simulink model "qn"  (R2025b)
settings: Solver=ode4  StartTime=0.0  StopTime=85  FixedStep=0.001  RelTol=1e-3
InitFcn:
  | % Codex-added defaults for qn controller parameters.
(part 2 of 2)

== system qn/11/control/eh uav pd10/Subsystem9 ==
  u : Inport
  MATLAB Function17 : MATLAB Function  TreatAsAtomicUnit=on
  y : Outport
  wires:
  u/1 -> MATLAB Function17/2(u)
  MATLAB Function17/1(y) -> y/1
  [falg] -> MATLAB Function17/1(flag)

== system qn/11/control/eh uav pd2/Subsystem1 ==
  u : Inport
  MATLAB Function15 : MATLAB Function  TreatAsAtomicUnit=on
  y : Outport
  wires:
  MATLAB Function15/1(y) -> y/1
  u/1 -> MATLAB Function15/2(u)
  [falg] -> MATLAB Function15/1(flag)

== system qn/11/control/eh uav pd2/Subsystem12 ==
  u : Inport
  MATLAB Function15 : MATLAB Function  TreatAsAtomicUnit=on
  y : Outport
  wires:
  MATLAB Function15/1(y) -> y/1
  u/1 -> MATLAB Function15/2(u)
  [falg] -> MATLAB Function15/1(flag)

== system qn/11/control/eh uav pd2/Subsystem2 ==
  u : Inport
  MATLAB Function15 : MATLAB Function  TreatAsAtomicUnit=on
  y : Outport
  wires:
  MATLAB Function15/1(y) -> y/1
  u/1 -> MATLAB Function15/2(u)
  [falg] -> MATLAB Function15/1(flag)

== system qn/11/control/eh uav pd3/Subsystem1 ==
  u : Inport
  MATLAB Function15 : MATLAB Function  TreatAsAtomicUnit=on
  y : Outport
  wires:
  MATLAB Function15/1(y) -> y/1
  u/1 -> MATLAB Function15/2(u)
  [falg] -> MATLAB Function15/1(flag)

== system qn/11/control/eh uav pd3/Subsystem12 ==
  u : Inport
  MATLAB Function15 : MATLAB Function  TreatAsAtomicUnit=on
  y : Outport
  wires:
  MATLAB Function15/1(y) -> y/1
  u/1 -> MATLAB Function15/2(u)
  [falg] -> MATLAB Function15/1(flag)

== system qn/11/control/eh uav pd3/Subsystem2 ==
  u : Inport
  MATLAB Function15 : MATLAB Function  TreatAsAtomicUnit=on
  y : Outport
  wires:
  MATLAB Function15/1(y) -> y/1
  u/1 -> MATLAB Function15/2(u)
  [falg] -> MATLAB Function15/1(flag)

== system qn/11/control/eh uav pd4/Subsystem1 ==
  u : Inport
  MATLAB Function15 : MATLAB Function  TreatAsAtomicUnit=on
  y : Outport
  wires:
  MATLAB Function15/1(y) -> y/1
  u/1 -> MATLAB Function15/2(u)
  [falg] -> MATLAB Function15/1(flag)

== system qn/11/control/eh uav pd4/Subsystem12 ==
  u : Inport
  MATLAB Function15 : MATLAB Function  TreatAsAtomicUnit=on
  y : Outport
  wires:
  MATLAB Function15/1(y) -> y/1
  u/1 -> MATLAB Function15/2(u)
  [falg] -> MATLAB Function15/1(flag)

== system qn/11/control/eh uav pd4/Subsystem2 ==
  u : Inport
  MATLAB Function15 : MATLAB Function  TreatAsAtomicUnit=on
  y : Outport
  wires:
  MATLAB Function15/1(y) -> y/1
  u/1 -> MATLAB Function15/2(u)
  [falg] -> MATLAB Function15/1(flag)

== system qn/11/control/eh uav pd5/Subsystem1 ==
  u : Inport
  MATLAB Function15 : MATLAB Function  TreatAsAtomicUnit=on
  y : Outport
  wires:
  MATLAB Function15/1(y) -> y/1
  u/1 -> MATLAB Function15/2(u)
  [falg] -> MATLAB Function15/1(flag)

== system qn/11/control/eh uav pd5/Subsystem12 ==
  u : Inport
  MATLAB Function15 : MATLAB Function  TreatAsAtomicUnit=on
  y : Outport
  wires:
  MATLAB Function15/1(y) -> y/1
  u/1 -> MATLAB Function15/2(u)
  [falg] -> MATLAB Function15/1(flag)

== system qn/11/control/eh uav pd5/Subsystem2 ==
  u : Inport
  MATLAB Function15 : MATLAB Function  TreatAsAtomicUnit=on
  y : Outport
  wires:
  MATLAB Function15/1(y) -> y/1
  u/1 -> MATLAB Function15/2(u)
  [falg] -> MATLAB Function15/1(flag)

== system qn/11/control/eh uav pd6/Subsystem1 ==
  u : Inport
  MATLAB Function17 : MATLAB Function  TreatAsAtomicUnit=on
  y : Outport
  wires:
  u/1 -> MATLAB Function17/2(u)
  MATLAB Function17/1(y) -> y/1
  [falg] -> MATLAB Function17/1(flag)

== system qn/11/control/eh uav pd6/Subsystem2 ==
  u : Inport
  MATLAB Function17 : MATLAB Function  TreatAsAtomicUnit=on
  y : Outport
  wires:
  u/1 -> MATLAB Function17/2(u)
  MATLAB Function17/1(y) -> y/1
  [falg] -> MATLAB Function17/1(flag)

== system qn/11/control/eh uav pd6/Subsystem9 ==
  u : Inport
  MATLAB Function17 : MATLAB Function  TreatAsAtomicUnit=on
  y : Outport
  wires:
  u/1 -> MATLAB Function17/2(u)
  MATLAB Function17/1(y) -> y/1
  [falg] -> MATLAB Function17/1(flag)

== system qn/11/control/eh uav pd7/Subsystem1 ==
  u : Inport
  MATLAB Function17 : MATLAB Function  TreatAsAtomicUnit=on
  y : Outport
  wires:
  u/1 -> MATLAB Function17/2(u)
  MATLAB Function17/1(y) -> y/1
  [falg] -> MATLAB Function17/1(flag)

== system qn/11/control/eh uav pd7/Subsystem2 ==
  u : Inport
  MATLAB Function17 : MATLAB Function  TreatAsAtomicUnit=on
  y : Outport
  wires:
  u/1 -> MATLAB Function17/2(u)
  MATLAB Function17/1(y) -> y/1
  [falg] -> MATLAB Function17/1(flag)

== system qn/11/control/eh uav pd7/Subsystem9 ==
  u : Inport
  MATLAB Function17 : MATLAB Function  TreatAsAtomicUnit=on
  y : Outport
  wires:
  u/1 -> MATLAB Function17/2(u)
  MATLAB Function17/1(y) -> y/1
  [falg] -> MATLAB Function17/1(flag)

== system qn/11/control/eh uav pd8/Subsystem1 ==
  u : Inport
  MATLAB Function17 : MATLAB Function  TreatAsAtomicUnit=on
  y : Outport
  wires:
  u/1 -> MATLAB Function17/2(u)
  MATLAB Function17/1(y) -> y/1
  [falg] -> MATLAB Function17/1(flag)

== system qn/11/control/eh uav pd8/Subsystem2 ==
  u : Inport
  MATLAB Function17 : MATLAB Function  TreatAsAtomicUnit=on
  y : Outport
  wires:
  u/1 -> MATLAB Function17/2(u)
  MATLAB Function17/1(y) -> y/1
  [falg] -> MATLAB Function17/1(flag)

== system qn/11/control/eh uav pd8/Subsystem9 ==
  u : Inport
  MATLAB Function17 : MATLAB Function  TreatAsAtomicUnit=on
  y : Outport
  wires:
  u/1 -> MATLAB Function17/2(u)
  MATLAB Function17/1(y) -> y/1
  [falg] -> MATLAB Function17/1(flag)

== system qn/11/control/eh uav pd9/Subsystem1 ==
  u : Inport
  MATLAB Function17 : MATLAB Function  TreatAsAtomicUnit=on
  y : Outport
  wires:
  u/1 -> MATLAB Function17/2(u)
  MATLAB Function17/1(y) -> y/1
  [falg] -> MATLAB Function17/1(flag)

== system qn/11/control/eh uav pd9/Subsystem2 ==
  u : Inport
  MATLAB Function17 : MATLAB Function  TreatAsAtomicUnit=on
  y : Outport
  wires:
  u/1 -> MATLAB Function17/2(u)
  MATLAB Function17/1(y) -> y/1
  [falg] -> MATLAB Function17/1(flag)

== system qn/11/control/eh uav pd9/Subsystem9 ==
  u : Inport
  MATLAB Function17 : MATLAB Function  TreatAsAtomicUnit=on
  y : Outport
  wires:
  u/1 -> MATLAB Function17/2(u)
  MATLAB Function17/1(y) -> y/1
  [falg] -> MATLAB Function17/1(flag)

== system qn/11/control/ex aav pd/Subsystem1 ==
  u : Inport
  MATLAB Function17 : MATLAB Function  TreatAsAtomicUnit=on
  y : Outport
  wires:
  u/1 -> MATLAB Function17/2(u)
  MATLAB Function17/1(y) -> y/1
  [falg] -> MATLAB Function17/1(flag)

== system qn/11/control/ex aav pd/Subsystem2 ==
  u : Inport
  MATLAB Function17 : MATLAB Function  TreatAsAtomicUnit=on
  y : Outport
  wires:
  u/1 -> MATLAB Function17/2(u)
  MATLAB Function17/1(y) -> y/1
  [falg] -> MATLAB Function17/1(flag)

== system qn/11/control/ex aav pd/Subsystem9 ==
  u : Inport
  MATLAB Function17 : MATLAB Function  TreatAsAtomicUnit=on
  y : Outport
  wires:
  u/1 -> MATLAB Function17/2(u)
  MATLAB Function17/1(y) -> y/1
  [falg] -> MATLAB Function17/1(flag)

== system qn/11/control/ey aav pd/Subsystem1 ==
  u : Inport
  MATLAB Function17 : MATLAB Function  TreatAsAtomicUnit=on
  y : Outport
  wires:
  u/1 -> MATLAB Function17/2(u)
  MATLAB Function17/1(y) -> y/1
  [falg] -> MATLAB Function17/1(flag)

== system qn/11/control/ey aav pd/Subsystem2 ==
  u : Inport
  MATLAB Function17 : MATLAB Function  TreatAsAtomicUnit=on
  y : Outport
  wires:
  u/1 -> MATLAB Function17/2(u)
  MATLAB Function17/1(y) -> y/1
  [falg] -> MATLAB Function17/1(flag)

== system qn/11/control/ey aav pd/Subsystem9 ==
  u : Inport
  MATLAB Function17 : MATLAB Function  TreatAsAtomicUnit=on
  y : Outport
  wires:
  u/1 -> MATLAB Function17/2(u)
  MATLAB Function17/1(y) -> y/1
  [falg] -> MATLAB Function17/1(flag)

== matlab function qn/11/control/Subsystem16/MATLAB Function17 ==
  data: flag input; u input; y output
function y = fcn(flag, u)
if flag==0
    y= u*0;
else
   y= u;
end

== matlab function qn/11/control/Subsystem17/MATLAB Function17 ==
  data: flag input; u input; y output
function y = fcn(flag, u)
if flag==0
    y= u*0;
else
   y= u;
end

== matlab function qn/11/control/Subsystem18/MATLAB Function17 ==
  data: flag input; u input; y output
function y = fcn(flag, u)
if flag==0
    y= u*0;
else
   y= u;
end

== matlab function qn/11/control/Subsystem19/MATLAB Function17 ==
  data: flag input; u input; y output
function y = fcn(flag, u)
if flag==0
    y= u*0;
else
   y= u;
end

== matlab function qn/Subsystem2/MATLAB Function8 ==
  data: dx input; xdn output; dy input; z input; yaw input; x1 input; y1 input; z1 input; xd input; yd input; hd input; ydn output; ex output; ey output; t2 output
function [xdn,ydn,ex,ey,t2]= fcn(dx,dy,z,yaw, x1,y1,z1,xd ,yd,hd)
ex=x1-xd;
ey=y1-yd;
[t2,~] = cart2pol(dx, dy);

 xdn=ex*cos(t2)+ey*sin(t2);
 ydn=ey*cos(t2)-ex*sin(t2);

== matlab function qn/11/control/Subsystem20/MATLAB Function17 ==
  data: flag input; u input; y output
function y = fcn(flag, u)
if flag==0
    y= u*0;
else
   y= u;
end

== matlab function qn/11/control/eh uav pd/Subsystem1/MATLAB Function15 ==
  data: flag input; u input; y output
function y = fcn(flag, u)
if flag==1
    y=u* 0;
else
   y= u;
end

== matlab function qn/11/control/Subsystem21/MATLAB Function17 ==
  data: flag input; u input; y output
function y = fcn(flag, u)
if flag==0
    y= u*0;
else
   y= u;
end

== matlab function qn/11/control/Subsystem22/MATLAB Function17 ==
  data: flag input; u input; y output
function y = fcn(flag, u)
if flag==0
    y= u*0;
else
   y= u;
end

== matlab function qn/11/control/Subsystem23/MATLAB Function17 ==
  data: flag input; u input; y output
function y = fcn(flag, u)
if flag==0
    y= u*0;
else
   y= u;
end

== matlab function qn/11/control/Subsystem24/MATLAB Function17 ==
  data: flag input; u input; y output
function y = fcn(flag, u)
if flag==0
    y= u*0;
else
   y= u;
end

== matlab function qn/11/control/Subsystem5/MATLAB Function15 ==
  data: flag input; u input; y output
function y = fcn(flag, u)
if flag==1
    y=u* 0;
else
   y= u;
end

== matlab function qn/Subsystem12/MATLAB Function ==
  data: xd output; yd output; x input; y input; x1 input; y1 input; h output
function [xd,yd,h] = fcn(x,y,x1,y1)


        xd=x;
        yd=y;
        h=-2;

== matlab function qn/11/plane modle/MATLAB Function ==
  data: wu1 input; T1 output; wu2 input; wp1 input; wp2 input; ws1 input; ws2 input; wf input; T2 output; Tf output; Tp1 output; Tp2 output; Ts1 output; Ts2 output; det1 input; det2 input; det3 input; det1 output; det2 output; det3 output
function [T1,T2,Tf,Tp1,Tp2,Ts1,Ts2,det1,det2,det3]  = fcn(wu1,wu2,wp1,wp2,ws1,ws2,wf,det1,det2,det3)
T1=wu1;
T2=wu2;
Tf=wf;
Tp1=wp1;
Tp2=wp2;
Ts1=ws1;
Ts2=ws2;

== matlab function qn/11/control/eh uav pd/Subsystem12/MATLAB Function15 ==
  data: flag input; u input; y output
function y = fcn(flag, u)
if flag==1
    y=u* 0;
else
   y= u;
end

== matlab function qn/11/plane modle/MATLAB Function1 ==
  data: M input; m output; m_d input; flag input
function m = fcn(M,m_d,flag)
if flag==0
m=M;
else if flag==1
m=M+m_d;
else
m=M*(flag+1);
end

end

== matlab function qn/11/plane modle/MATLAB Function2 ==
  data: jxx input; J output; jyy input; jzz input; jxx_d input; jyy_d input; jzz_d input; flag input
function J = fcn(jxx,jyy,jzz,jxx_d,jyy_d,jzz_d,flag)
if flag==0
J=[jxx 0 0;0 jyy 0; 0 0 jzz];
else if flag==1
J=[jxx 0 0;0 jyy 0; 0 0 jzz]+[jxx_d 0 0;0 jyy_d 0; 0 0 jzz_d];
else
J=[jxx 0 0;0 jyy 0; 0 0 jzz]*(flag+1);
end

end

== matlab function qn/Subsystem/MATLAB Function ==
  data: t input; h output
function h = fcn(t)
h=-5*cos(t);

== matlab function qn/Subsystem12/MATLAB Function1 ==
  data: x input; y input; yaw input; dx input; dy input; X input; xd input; xdn output; yd input; ydn output; t2 output; dxdn output; dydn output; yaw output; X output; ex output; ey output
function [xdn,ydn,t2,dxdn,dydn,yaw,X,ex,ey] = fcn( x,y,yaw,dx,dy,X, xd,yd)

ex=x-xd;
ey=y-yd;
t2=atan2(-ey,-ex);

 xdn=ex*cos(yaw)+ey*sin(yaw);
 ydn=ey*cos(yaw)-ex*sin(yaw);
 dxdn=dx*cos(yaw)+dy*sin(yaw);
 dydn=dy*cos(yaw)-dx*sin(yaw);

== matlab function qn/11/control/Subsystem1/MATLAB Function15 ==
  data: flag input; u input; y output
function y = fcn(flag, u)
if flag==1
    y=u* 0;
else
   y= u;
end

== matlab function qn/11/control/Subsystem3/MATLAB Function15 ==
  data: flag input; u input; y output
function y = fcn(flag, u)
if flag==1
    y=u* 0;
else
   y= u;
end

== matlab function qn/11/control/Subsystem29/MATLAB Function15 ==
  data: flag input; u input; y output
function y = fcn(flag, u)
if flag==1
    y=u* 0;
else
   y= u;
end

== matlab function qn/11/control/Subsystem32/MATLAB Function15 ==
  data: flag input; u input; y output
function y = fcn(flag, u)
if flag==1
    y=u* 0;
else
   y= u;
end

== matlab function qn/11/control/eh uav pd/Subsystem2/MATLAB Function15 ==
  data: flag input; u input; y output
function y = fcn(flag, u)
if flag==1
    y=u* 0;
else
   y= u;
end

== matlab function qn/11/control/Subsystem33/MATLAB Function15 ==
  data: flag input; u input; y output
function y = fcn(flag, u)
if flag==1
    y=u* 0;
else
   y= u;
end

== matlab function qn/11/control/Subsystem36/MATLAB Function15 ==
  data: flag input; u input; y output
function y = fcn(flag, u)
if flag==1
    y=u* 0;
else
   y= u;
end

== matlab function qn/11/control/Subsystem38/MATLAB Function15 ==
  data: flag input; u input; y output
function y = fcn(flag, u)
if flag==1
    y=u* 0;
else
   y= u;
end

== matlab function qn/11/control/Subsystem39/MATLAB Function15 ==
  data: flag input; u input; y output
function y = fcn(flag, u)
if flag==1
    y=u* 0;
else
   y= u;
end

== matlab function qn/11/control/Subsystem41/MATLAB Function15 ==
  data: flag input; u input; y output
function y = fcn(flag, u)
if flag==1
    y=u* 0;
else
   y= u;
end

== matlab function qn/11/control/eh uav pd/pd1 ==
  data: x input; u output; r input; fxp input; b input; x1 input; x2 input; k1 input; k2 input
function u = fcn(x,r,fxp,b,x1,x2,k1,k2)
% z1=x1-r;
% % z2=x2
z2=x(2);
z1=x(1)-r;
% k1=wc*wc;
% k2=wc*2;
u=(-k1*z1-k2*z2-fxp)/b;

== matlab function qn/Subsystem/MATLAB Function3 ==
  data: dx output; dy output; v input; t input; X output
function [dx,dy,X]= fcn(v,t)
dx=v*cos(t);
dy=v*sin(t);
X=atan2(dy,dx);

== matlab function qn/11/control/eh uav pd2/Subsystem1/MATLAB Function15 ==
  data: flag input; u input; y output
function y = fcn(flag, u)
if flag==1
    y=u* 0;
else
   y= u;
end

== matlab function qn/11/ earth environment/MATLAB Function ==
  data: v_x input; u_w output; v_y input; v_z input; v_w output; w_w output; e1 input; e2 input; e3 input; e0 input
function [u_w,v_w,w_w] = fcn(v_x,v_y,v_z,e1,e2,e3,e0)
u_w=v_x*(e1*e1+e0*e0-e2*e2-e3*e3)+2*v_y*(e1*e2-e3*e0)+2*v_z*(e1*e3+e2*e0);
v_w=2*v_x*(e1*e2+e3*e0)+v_y*(e2*e2+e0*e0-e1*e1-e3*e3)+2*v_z*(e2*e3-e1*e0);
w_w=2*v_x*(e1*e3-e2*e0)+2*v_y*(e2*e3+e1*e0)+v_z*(e3*e3+e0*e0-e2*e2-e1*e1);

== matlab function qn/11/control/eh uav pd2/Subsystem12/MATLAB Function15 ==
  data: flag input; u input; y output
function y = fcn(flag, u)
if flag==1
    y=u* 0;
else
   y= u;
end

== matlab function qn/11/control/eh uav pd2/Subsystem2/MATLAB Function15 ==
  data: flag input; u input; y output
function y = fcn(flag, u)
if flag==1
    y=u* 0;
else
   y= u;
end

== matlab function qn/11/control/eh uav pd2/pd1 ==
  data: x input; u output; r input; fxp input; b input; x1 input; x2 input; k1 input; k2 input
function u = fcn(x,r,fxp,b,x1,x2,k1,k2)
% z1=x1-r;
% % z2=x2
z2=x(2);
z1=x(1)-r;
% k1=wc*wc;
% k2=wc*2;
u=(-k1*z1-k2*z2-fxp)/b;

== matlab function qn/11/control/eh uav pd3/MATLAB Function9 ==
  data: dx output; ut input; b1 input; x input size=[2 1]; q input; W1 input size=[1 7]; dW1 output; fxp output; w0 input; F1 input
function [dx,dW1,fxp] = fcn(ut,b1,x,q,W1,w0,F1)

%%
h=zeros(1,7);

%%
K1=2*w0;K2=w0*w0;
%  F1=w0^3;
%%
c1=1/3*[-3 -2 -1 0 1 2 3];
c2=2/3*[-3 -2 -1 0 1 2 3];
c=[c1;c2];
b=5;
xp=x';
ye=(q-x(1));
%%
for j=1:1:7
    h(j)=exp(-norm(xp-c(:,j))^2/(2*b^2));
end

k1=0.001;
% k1=0;k2=0;
dW1=F1*h*ye-k1*F1*abs(ye)*W1;

fxp=W1*h';
%%


y=q;
A=[0 1;0 0];
b=[0 1]';
C=[1 0];
K=[K1 K2]';

ye=y-x(1);
D=0;
v=-D*sign(ye);

dx=A*x+b*(fxp+b1*ut-v)+K*(y-C*x);

== matlab function qn/11/control/eh uav pd3/Subsystem1/MATLAB Function15 ==
  data: flag input; u input; y output
function y = fcn(flag, u)
if flag==1
    y=u* 0;
else
   y= u;
end

== matlab function qn/11/control/eh uav pd3/Subsystem12/MATLAB Function15 ==
  data: flag input; u input; y output
function y = fcn(flag, u)
if flag==1
    y=u* 0;
else
   y= u;
end

== matlab function qn/11/control/eh uav pd3/Subsystem2/MATLAB Function15 ==
  data: flag input; u input; y output
function y = fcn(flag, u)
if flag==1
    y=u* 0;
else
   y= u;
end

== matlab function qn/11/control/eh uav pd3/pd1 ==
  data: x input; u output; r input; fxp input; b input; x1 input; x2 input; k1 input; k2 input
function u = fcn(x,r,fxp,b,x1,x2,k1,k2)
% z1=x1-r;
% % z2=x2
z2=x(2);
z1=x(1)-r;
% k1=wc*wc;
% k2=wc*2;
u=(-k1*z1-k2*z2-fxp)/b;

== matlab function qn/11/control/eh uav pd4/MATLAB Function9 ==
  data: dx output; ut input; b1 input; x input size=[2 1]; q input; W1 input size=[1 7]; dW1 output; fxp output; w0 input; F1 input
function [dx,dW1,fxp] = fcn(ut,b1,x,q,W1,w0,F1)

%%
h=zeros(1,7);

%%
K1=2*w0;K2=w0*w0;
%  F1=w0^3;
%%
c1=1/3*[-3 -2 -1 0 1 2 3];
c2=2/3*[-3 -2 -1 0 1 2 3];
c=[c1;c2];
b=5;
xp=x';
ye=(q-x(1));
%%
for j=1:1:7
    h(j)=exp(-norm(xp-c(:,j))^2/(2*b^2));
end

k1=0.001;
% k1=0;k2=0;
dW1=F1*h*ye-k1*F1*abs(ye)*W1;

fxp=W1*h';
%%


y=q;
A=[0 1;0 0];
b=[0 1]';
C=[1 0];
K=[K1 K2]';

ye=y-x(1);
D=0;
v=-D*sign(ye);

dx=A*x+b*(fxp+b1*ut-v)+K*(y-C*x);

== matlab function qn/11/control/eh uav pd6/MATLAB Function9 ==
  data: dx output; ut input; b1 input; x input size=[2 1]; q input; W1 input size=[1 7]; dW1 output; fxp output; w0 input; F1 input
function [dx,dW1,fxp] = fcn(ut,b1,x,q,W1,w0,F1)

%%
h=zeros(1,7);

%%
K1=2*w0;K2=w0*w0;
%  F1=w0^3;
%%
c1=1/3*[-3 -2 -1 0 1 2 3];
c2=2/3*[-3 -2 -1 0 1 2 3];
c=[c1;c2];
b=5;
xp=x';
ye=(q-x(1));
%%
for j=1:1:7
    h(j)=exp(-norm(xp-c(:,j))^2/(2*b^2));
end

k1=0.001;
% k1=0;k2=0;
dW1=F1*h*ye-k1*F1*abs(ye)*W1;

fxp=W1*h';
%%


y=q;
A=[0 1;0 0];
b=[0 1]';
C=[1 0];
K=[K1 K2]';

ye=y-x(1);
D=0;
v=-D*sign(ye);

dx=A*x+b*(fxp+b1*ut-v)+K*(y-C*x);

== matlab function qn/11/control/eh uav pd4/Subsystem1/MATLAB Function15 ==
  data: flag input; u input; y output
function y = fcn(flag, u)
if flag==1
    y=u* 0;
else
   y= u;
end

== matlab function qn/11/control/eh uav pd4/Subsystem12/MATLAB Function15 ==
  data: flag input; u input; y output
function y = fcn(flag, u)
if flag==1
    y=u* 0;
else
   y= u;
end

== matlab function qn/11/control/MATLAB Function7 ==
  data: y output; r input; e output; yaw input
function [y,e]  = fcn(r,yaw)
% r=0.2*u;
e=yaw-r;
% if e>pi
%     s1=mod(e+pi,2*pi)-pi;
% elseif e<-pi
%     s1=mod(e-pi,-2*pi);
% else
%     s1=e;
% end
s1=mod(e+pi,2*pi)-pi;
y=s1;

== matlab function qn/11/control/eh uav pd6/Subsystem1/MATLAB Function17 ==
  data: flag input; u input; y output
function y = fcn(flag, u)
if flag==0
    y= u*0;
else
   y= u;
end

== matlab function qn/11/control/eh uav pd6/Subsystem9/MATLAB Function17 ==
  data: flag input; u input; y output
function y = fcn(flag, u)
if flag==0
    y= u*0;
else
   y= u;
end

== matlab function qn/11/control/eh uav pd6/Subsystem2/MATLAB Function17 ==
  data: flag input; u input; y output
function y = fcn(flag, u)
if flag==0
    y= u*0;
else
   y= u;
end

== matlab function qn/11/control/eh uav pd6/pd1 ==
  data: x input; u output; r input; fxp input; b input; x1 input; x2 input; k1 input; k2 input
function u = fcn(x,r,fxp,b,x1,x2,k1,k2)
% z1=x1-r;
% % z2=x2
z2=x(2);
z1=x(1)-r;
% k1=wc*wc;
% k2=wc*2;
u=(-k1*z1-k2*z2-fxp)/b;

== matlab function qn/11/control/eh uav pd4/Subsystem2/MATLAB Function15 ==
  data: flag input; u input; y output
function y = fcn(flag, u)
if flag==1
    y=u* 0;
else
   y= u;
end

== matlab function qn/11/control/eh uav pd4/pd1 ==
  data: x input; u output; r input; fxp input; b input; x1 input; x2 input; k1 input; k2 input
function u = fcn(x,r,fxp,b,x1,x2,k1,k2)
% z1=x1-r;
% % z2=x2
z2=x(2);
z1=x(1)-r;
% k1=wc*wc;
% k2=wc*2;
u=(-k1*z1-k2*z2-fxp)/b;

== matlab function qn/11/control/eh uav pd1/MATLAB Function9 ==
  data: dx output; ut input; b1 input; x input size=[2 1]; q input; W1 input size=[1 7]; dW1 output; fxp output; w0 input; F1 input
function [dx,dW1,fxp] = fcn(ut,b1,x,q,W1,w0,F1)

%%
h=zeros(1,7);

%%
K1=2*w0;K2=w0*w0;
%  F1=w0^3;
%%
c1=1/3*[-3 -2 -1 0 1 2 3];
c2=2/3*[-3 -2 -1 0 1 2 3];
c=[c1;c2];
b=5;
xp=x';
ye=(q-x(1));
%%
for j=1:1:7
    h(j)=exp(-norm(xp-c(:,j))^2/(2*b^2));
end

k1=0.001;
% k1=0;k2=0;
dW1=F1*h*ye-k1*F1*abs(ye)*W1;

fxp=W1*h';
%%


y=q;
A=[0 1;0 0];
b=[0 1]';
C=[1 0];
K=[K1 K2]';

ye=y-x(1);
D=0;
v=-D*sign(ye);

dx=A*x+b*(fxp+b1*ut-v)+K*(y-C*x);

== matlab function qn/11/control/eh uav pd1/Subsystem1/MATLAB Function15 ==
  data: flag input; u input; y output
function y = fcn(flag, u)
if flag==1
    y=u* 0;
else
   y= u;
end

== matlab function qn/11/control/eh uav pd1/Subsystem12/MATLAB Function15 ==
  data: flag input; u input; y output
function y = fcn(flag, u)
if flag==1
    y=u* 0;
else
   y= u;
end

== matlab function qn/11/control/eh uav pd1/Subsystem2/MATLAB Function15 ==
  data: flag input; u input; y output
function y = fcn(flag, u)
if flag==1
    y=u* 0;
else
   y= u;
end

== matlab function qn/11/control/eh uav pd1/pd1 ==
  data: x input; u output; r input; fxp input; b input; x1 input; x2 input; k1 input; k2 input
function u = fcn(x,r,fxp,b,x1,x2,k1,k2)
% z1=x1-r;
% % z2=x2
z2=x(2);
z1=x(1)-r;
% k1=wc*wc;
% k2=wc*2;
u=(-k1*z1-k2*z2-fxp)/b;

== matlab function qn/11/control/eh uav pd5/MATLAB Function9 ==
  data: dx output; ut input; b1 input; x input size=[2 1]; q input; W1 input size=[1 7]; dW1 output; fxp output; w0 input; F1 input
function [dx,dW1,fxp] = fcn(ut,b1,x,q,W1,w0,F1)

%%
h=zeros(1,7);

%%
K1=2*w0;K2=w0*w0;
%  F1=w0^3;
%%
c1=1/3*[-3 -2 -1 0 1 2 3];
c2=2/3*[-3 -2 -1 0 1 2 3];
c=[c1;c2];
b=5;
xp=x';
ye=(q-x(1));
%%
for j=1:1:7
    h(j)=exp(-norm(xp-c(:,j))^2/(2*b^2));
end

k1=0.001;
% k1=0;k2=0;
dW1=F1*h*ye-k1*F1*abs(ye)*W1;

fxp=W1*h';
%%


y=q;
A=[0 1;0 0];
b=[0 1]';
C=[1 0];
K=[K1 K2]';

ye=y-x(1);
D=0;
v=-D*sign(ye);

dx=A*x+b*(fxp+b1*ut-v)+K*(y-C*x);

== matlab function qn/11/control/eh uav pd5/Subsystem1/MATLAB Function15 ==
  data: flag input; u input; y output
function y = fcn(flag, u)
if flag==1
    y=u* 0;
else
   y= u;
end

== matlab function qn/11/control/eh uav pd5/Subsystem12/MATLAB Function15 ==
  data: flag input; u input; y output
function y = fcn(flag, u)
if flag==1
    y=u* 0;
else
   y= u;
end

== matlab function qn/11/control/eh uav pd5/Subsystem2/MATLAB Function15 ==
  data: flag input; u input; y output
function y = fcn(flag, u)
if flag==1
    y=u* 0;
else
   y= u;
end

== matlab function qn/11/control/eh uav pd5/pd1 ==
  data: x input; u output; r input; fxp input; b input; x1 input; x2 input; k1 input; k2 input
function u = fcn(x,r,fxp,b,x1,x2,k1,k2)
% z1=x1-r;
% % z2=x2
z2=x(2);
z1=x(1)-r;
% k1=wc*wc;
% k2=wc*2;
u=(-k1*z1-k2*z2-fxp)/b;

== matlab function qn/11/control/eh uav pd7/MATLAB Function9 ==
  data: dx output; ut input; b1 input; x input size=[2 1]; q input; W1 input size=[1 7]; dW1 output; fxp output; w0 input; F1 input
function [dx,dW1,fxp] = fcn(ut,b1,x,q,W1,w0,F1)

%%
h=zeros(1,7);

%%
K1=2*w0;K2=w0*w0;
%  F1=w0^3;
%%
c1=1/3*[-3 -2 -1 0 1 2 3];
c2=2/3*[-3 -2 -1 0 1 2 3];
c=[c1;c2];
b=5;
xp=x';
ye=(q-x(1));
%%
for j=1:1:7
    h(j)=exp(-norm(xp-c(:,j))^2/(2*b^2));
end

k1=0.001;
% k1=0;k2=0;
dW1=F1*h*ye-k1*F1*abs(ye)*W1;

fxp=W1*h';
%%


y=q;
A=[0 1;0 0];
b=[0 1]';
C=[1 0];
K=[K1 K2]';

ye=y-x(1);
D=0;
v=-D*sign(ye);

dx=A*x+b*(fxp+b1*ut-v)+K*(y-C*x);

== matlab function qn/11/control/eh uav pd7/Subsystem1/MATLAB Function17 ==
  data: flag input; u input; y output
function y = fcn(flag, u)
if flag==0
    y= u*0;
else
   y= u;
end

== matlab function qn/11/control/eh uav pd7/Subsystem2/MATLAB Function17 ==
  data: flag input; u input; y output
function y = fcn(flag, u)
if flag==0
    y= u*0;
else
   y= u;
end

== matlab function qn/11/control/eh uav pd9/MATLAB Function9 ==
  data: dx output; ut input; b1 input; x input size=[2 1]; q input; W1 input size=[1 7]; dW1 output; fxp output; w0 input; F1 input
function [dx,dW1,fxp] = fcn(ut,b1,x,q,W1,w0,F1)

%%
h=zeros(1,7);

%%
K1=2*w0;K2=w0*w0;
%  F1=w0^3;
%%
c1=1/3*[-3 -2 -1 0 1 2 3];
c2=2/3*[-3 -2 -1 0 1 2 3];
c=[c1;c2];
b=5;
xp=x';
ye=(q-x(1));
%%
for j=1:1:7
    h(j)=exp(-norm(xp-c(:,j))^2/(2*b^2));
end

k1=0.001;
% k1=0;k2=0;
dW1=F1*h*ye-k1*F1*abs(ye)*W1;

fxp=W1*h';
%%


y=q;
A=[0 1;0 0];
b=[0 1]';
C=[1 0];
K=[K1 K2]';

ye=y-x(1);
D=0;
v=-D*sign(ye);

dx=A*x+b*(fxp+b1*ut-v)+K*(y-C*x);

== matlab function qn/11/control/eh uav pd9/Subsystem1/MATLAB Function17 ==
  data: flag input; u input; y output
function y = fcn(flag, u)
if flag==0
    y= u*0;
else
   y= u;
end

== matlab function qn/11/control/eh uav pd9/Subsystem2/MATLAB Function17 ==
  data: flag input; u input; y output
function y = fcn(flag, u)
if flag==0
    y= u*0;
else
   y= u;
end

== matlab function qn/11/control/eh uav pd9/Subsystem9/MATLAB Function17 ==
  data: flag input; u input; y output
function y = fcn(flag, u)
if flag==0
    y= u*0;
else
   y= u;
end

== matlab function qn/11/control/eh uav pd9/pd1 ==
  data: x input; u output; r input; fxp input; b input; x1 input; x2 input; k1 input; k2 input
function u = fcn(x,r,fxp,b,x1,x2,k1,k2)
% z1=x1-r;
% % z2=x2
z2=x(2);
z1=x(1)-r;
% k1=wc*wc;
% k2=wc*2;
u=(-k1*z1-k2*z2-fxp)/b;

== matlab function qn/11/control/eh uav pd7/Subsystem9/MATLAB Function17 ==
  data: flag input; u input; y output
function y = fcn(flag, u)
if flag==0
    y= u*0;
else
   y= u;
end

== matlab function qn/11/control/eh uav pd7/pd1 ==
  data: x input; u output; r input; fxp input; b input; x1 input; x2 input; k1 input; k2 input
function u = fcn(x,r,fxp,b,x1,x2,k1,k2)
% z1=x1-r;
% % z2=x2
z2=x(2);
z1=x(1)-r;
% k1=wc*wc;
% k2=wc*2;
u=(-k1*z1-k2*z2-fxp)/b;

== matlab function qn/11/control/eh uav pd10/MATLAB Function9 ==
  data: dx output; ut input; b1 input; x input size=[2 1]; q input; W1 input size=[1 7]; dW1 output; fxp output; w0 input; F1 input
function [dx,dW1,fxp] = fcn(ut,b1,x,q,W1,w0,F1)

%%
h=zeros(1,7);

%%
K1=2*w0;K2=w0*w0;
%  F1=w0^3;
%%
c1=1/3*[-3 -2 -1 0 1 2 3];
c2=2/3*[-3 -2 -1 0 1 2 3];
c=[c1;c2];
b=5;
xp=x';
ye=(q-x(1));
%%
for j=1:1:7
    h(j)=exp(-norm(xp-c(:,j))^2/(2*b^2));
end

k1=0.001;
% k1=0;k2=0;
dW1=F1*h*ye-k1*F1*abs(ye)*W1;

fxp=W1*h';
%%


y=q;
A=[0 1;0 0];
b=[0 1]';
C=[1 0];
K=[K1 K2]';

ye=y-x(1);
D=0;
v=-D*sign(ye);

dx=A*x+b*(fxp+b1*ut-v)+K*(y-C*x);

== matlab function qn/11/control/eh uav pd10/Subsystem1/MATLAB Function17 ==
  data: flag input; u input; y output
function y = fcn(flag, u)
if flag==0
    y= u*0;
else
   y= u;
end

== matlab function qn/11/control/eh uav pd10/Subsystem2/MATLAB Function17 ==
  data: flag input; u input; y output
function y = fcn(flag, u)
if flag==0
    y= u*0;
else
   y= u;
end

== matlab function qn/11/control/eh uav pd10/Subsystem9/MATLAB Function17 ==
  data: flag input; u input; y output
function y = fcn(flag, u)
if flag==0
    y= u*0;
else
   y= u;
end

== matlab function qn/11/control/eh uav pd10/pd1 ==
  data: x input; u output; r input; fxp input; b input; x1 input; x2 input; k1 input; k2 input
function u = fcn(x,r,fxp,b,x1,x2,k1,k2)
% z1=x1-r;
% % z2=x2
z2=x(2);
z1=x(1)-r;
% k1=wc*wc;
% k2=wc*2;
u=(-k1*z1-k2*z2-fxp)/b;

== matlab function qn/11/control/eh uav pd8/MATLAB Function9 ==
  data: dx output; ut input; b1 input; x input size=[2 1]; q input; W1 input size=[1 7]; dW1 output; fxp output; w0 input; F1 input
function [dx,dW1,fxp] = fcn(ut,b1,x,q,W1,w0,F1)

%%
h=zeros(1,7);

%%
K1=2*w0;K2=w0*w0;
%  F1=w0^3;
%%
c1=1/3*[-3 -2 -1 0 1 2 3];
c2=2/3*[-3 -2 -1 0 1 2 3];
c=[c1;c2];
b=5;
xp=x';
ye=(q-x(1));
%%
for j=1:1:7
    h(j)=exp(-norm(xp-c(:,j))^2/(2*b^2));
end

k1=0.001;
% k1=0;k2=0;
dW1=F1*h*ye-k1*F1*abs(ye)*W1;

fxp=W1*h';
%%


y=q;
A=[0 1;0 0];
b=[0 1]';
C=[1 0];
K=[K1 K2]';

ye=y-x(1);
D=0;
v=-D*sign(ye);

dx=A*x+b*(fxp+b1*ut-v)+K*(y-C*x);

== matlab function qn/11/control/eh uav pd8/Subsystem1/MATLAB Function17 ==
  data: flag input; u input; y output
function y = fcn(flag, u)
if flag==0
    y= u*0;
else
   y= u;
end

== matlab function qn/11/control/eh uav pd8/Subsystem2/MATLAB Function17 ==
  data: flag input; u input; y output
function y = fcn(flag, u)
if flag==0
    y= u*0;
else
   y= u;
end

== matlab function qn/11/control/ex aav pd/MATLAB Function9 ==
  data: dx output; ut input; b1 input; x input size=[2 1]; q input; W1 input size=[1 7]; dW1 output; fxp output; w0 input; F1 input
function [dx,dW1,fxp] = fcn(ut,b1,x,q,W1,w0,F1)

%%
h=zeros(1,7);

%%
K1=2*w0;K2=w0*w0;
%  F1=w0^3;
%%
c1=1/3*[-3 -2 -1 0 1 2 3];
c2=2/3*[-3 -2 -1 0 1 2 3];
c=[c1;c2];
b=5;
xp=x';
ye=(q-x(1));
%%
for j=1:1:7
    h(j)=exp(-norm(xp-c(:,j))^2/(2*b^2));
end

k1=0.001;
% k1=0;k2=0;
dW1=F1*h*ye-k1*F1*abs(ye)*W1;

fxp=W1*h';
%%


y=q;
A=[0 1;0 0];
b=[0 1]';
C=[1 0];
K=[K1 K2]';

ye=y-x(1);
D=0;
v=-D*sign(ye);

dx=A*x+b*(fxp+b1*ut-v)+K*(y-C*x);

== matlab function qn/11/control/eh uav pd8/Subsystem9/MATLAB Function17 ==
  data: flag input; u input; y output
function y = fcn(flag, u)
if flag==0
    y= u*0;
else
   y= u;
end

== matlab function qn/11/control/eh uav pd8/pd1 ==
  data: x input; u output; r input; fxp input; b input; x1 input; x2 input; k1 input; k2 input
function u = fcn(x,r,fxp,b,x1,x2,k1,k2)
% z1=x1-r;
% % z2=x2
z2=x(2);
z1=x(1)-r;
% k1=wc*wc;
% k2=wc*2;
u=(-k1*z1-k2*z2-fxp)/b;

== matlab function qn/11/control/ex aav pd/Subsystem1/MATLAB Function17 ==
  data: flag input; u input; y output
function y = fcn(flag, u)
if flag==0
    y= u*0;
else
   y= u;
end

== matlab function qn/11/control/ex aav pd/Subsystem9/MATLAB Function17 ==
  data: flag input; u input; y output
function y = fcn(flag, u)
if flag==0
    y= u*0;
else
   y= u;
end

== matlab function qn/11/control/ex aav pd/Subsystem2/MATLAB Function17 ==
  data: flag input; u input; y output
function y = fcn(flag, u)
if flag==0
    y= u*0;
else
   y= u;
end

== matlab function qn/11/control/ex aav pd/pd1 ==
  data: x input; u output; r input; fxp input; wc input; b input; x1 input; x2 input
function u = fcn(x,r,fxp,wc,b,x1,x2)
% z1=x1-r;
% z2=x2
z2=x(2);
z1=x(1)-r;
k1=wc*wc;
k2=wc*2;
u=(-k1*z1-k2*z2-fxp)/b;
% u=(-k1*(0.5*sign(z1)*abs(z1)^0.99+0.5*sign(z1)*abs(z1)^1.01)-k12*z2-fxp)/b;

== matlab function qn/MATLAB Function ==
  data: x1 input; ex output; y1 input; z1 input; xd input; yd input; zd input; ey output; ez output; rmse output
function [ex,ey,ez,rmse] = fcn(x1,y1,z1,xd,yd,zd)
ex=x1-xd;
ey=y1-yd;
ez=z1-zd;
rmse=sqrt(ex*ex+ey*ey+ez*ez);

== matlab function qn/11/control/eh uav pd2/MATLAB Function9 ==
  data: dx output; ut input; b1 input; x input size=[2 1]; q input; W1 input size=[1 7]; dW1 output; fxp output; w0 input; F1 input
function [dx,dW1,fxp] = fcn(ut,b1,x,q,W1,w0,F1)

%%
h=zeros(1,7);

%%
K1=2*w0;K2=w0*w0;
%  F1=w0^3;
%%
c1=1/3*[-3 -2 -1 0 1 2 3];
c2=2/3*[-3 -2 -1 0 1 2 3];
c=[c1;c2];
b=5;
xp=x';
ye=(q-x(1));
%%
for j=1:1:7
    h(j)=exp(-norm(xp-c(:,j))^2/(2*b^2));
end

k1=0.001;
% k1=0;k2=0;
dW1=F1*h*ye-k1*F1*abs(ye)*W1;

fxp=W1*h';
%%


y=q;
A=[0 1;0 0];
b=[0 1]';
C=[1 0];
K=[K1 K2]';

ye=y-x(1);
D=0;
v=-D*sign(ye);

dx=A*x+b*(fxp+b1*ut-v)+K*(y-C*x);

== matlab function qn/11/control/ey aav pd/MATLAB Function9 ==
  data: dx output; ut input; b1 input; x input size=[2 1]; q input; W1 input size=[1 7]; dW1 output; fxp output; w0 input; F1 input
function [dx,dW1,fxp] = fcn(ut,b1,x,q,W1,w0,F1)

%%
h=zeros(1,7);

%%
K1=2*w0;K2=w0*w0;
%  F1=w0^3;
%%
c1=1/3*[-3 -2 -1 0 1 2 3];
c2=2/3*[-3 -2 -1 0 1 2 3];
c=[c1;c2];
b=5;
xp=x';
ye=(q-x(1));
%%
for j=1:1:7
    h(j)=exp(-norm(xp-c(:,j))^2/(2*b^2));
end

k1=0.001;
% k1=0;k2=0;
dW1=F1*h*ye-k1*F1*abs(ye)*W1;

fxp=W1*h';
%%


y=q;
A=[0 1;0 0];
b=[0 1]';
C=[1 0];
K=[K1 K2]';

ye=y-x(1);
D=0;
v=-D*sign(ye);

dx=A*x+b*(fxp+b1*ut-v)+K*(y-C*x);

== matlab function qn/11/control/ey aav pd/Subsystem1/MATLAB Function17 ==
  data: flag input; u input; y output
function y = fcn(flag, u)
if flag==0
    y= u*0;
else
   y= u;
end

== matlab function qn/11/control/ey aav pd/Subsystem9/MATLAB Function17 ==
  data: flag input; u input; y output
function y = fcn(flag, u)
if flag==0
    y= u*0;
else
   y= u;
end

== matlab function qn/11/control/ey aav pd/Subsystem2/MATLAB Function17 ==
  data: flag input; u input; y output
function y = fcn(flag, u)
if flag==0
    y= u*0;
else
   y= u;
end

== matlab function qn/11/control/ey aav pd/pd1 ==
  data: x input; u output; r input; fxp input; wc input; b input; x1 input; x2 input
function u = fcn(x,r,fxp,wc,b,x1,x2)
% z1=x1-r;
% z2=x2
z2=x(2);
z1=x(1)-r;
k1=wc*wc;
k2=wc*2;
u=(-k1*z1-k2*z2-fxp)/b;
% u=(-k1*(0.5*sign(z1)*abs(z1)^0.99+0.5*sign(z1)*abs(z1)^1.01)-k12*z2-fxp)/b;

== matlab function qn/11/ earth environment/air ==
  data: input_h input; rou output
function rou = fcn(input_h)
h=input_h+65;
rho0=1.225;T0=288.15;
if h<=11000
    T=T0-0.0065*h;
    rou=rho0*(T/T0)^4.25588;
elseif h>11000&&h<=20000
    T=216.65;
    rou=0.36392*exp((-h+11000)/6341.62);
else
    T=216.65+0.001*(h-20000);
    rou=0.088035*(T/216.65)^-35.1632;
end

== matlab function qn/11/MATLAB Function3 ==
  data: h input; flag output; hg input
function flag = fcn(h,hg)
if h>=0.5*hg
    flag=0;
else if h<=-0.5*hg
        flag=1;
else
    flag=0.5-h/hg;
end
end

== matlab function qn/11/ODE/12ODE ==
  settings: sampleTime=13
  data: dX input; ddX output; e0 input; e1 input; e2 input; e3 input; g input; J input; m input; F input; dx output size=1; dy output size=1; dh output size=1; de0 output size=1; de1 output size=1; de2 output size=1; de3 output size=1; DCM output; bigM output; bigC output
function [ddX,dx,dy,dh,de0,de1,de2,de3,DCM,bigM,bigC] = fcn(dX,e0,e1,e2,e3, g,J,m,F)
u=dX(1);
v=dX(2);
w=dX(3);
p=dX(4);
q=dX(5);
r=dX(6);

MM=diag([m m m]);
Z=zeros(3,3);
X=Z;
bigM=[MM,X;X',J];
w1=[0 -r q;
    r 0 -p;
    -q p 0];
bigC=[MM*w1,Z;Z w1*J];
%%


%% 下为正

G=[m*g*2*(e1*e3-e2*e0);
   2*m*g*(e2*e3+e1*e0);
   m*g*(e3*e3+e0*e0-e1*e1-e2*e2);
   0;0;0];

bigF=F+G;
ddX=(bigM)\(bigF-bigC*dX);

%%
dx=u*(e1*e1+e0*e0-e2*e2-e3*e3)+2*v*(e1*e2-e3*e0)+2*w*(e1*e3+e2*e0);
dy=2*u*(e1*e2+e3*e0)+v*(e2*e2+e0*e0-e1*e1-e3*e3)+2*w*(e2*e3-e1*e0);
dh=-2*u*(e1*e3-e2*e0)-2*v*(e2*e3+e1*e0)-w*(e3*e3+e0*e0-e2*e2-e1*e1);
%%
de0=-0.5*(p*e1+q*e2+r*e3);
de1=0.5*(p*e0+r*e2-q*e3);
de2=0.5*(q*e0-r*e1+p*e3);
de3=0.5*(r*e0+q*e1-p*e2);
%%
DCM=[(e1*e1+e0*e0-e2*e2-e3*e3),2*(e1*e2-e3*e0),2*(e1*e3+e2*e0);
     2*(e1*e2+e3*e0), (e2*e2+e0*e0-e1*e1-e3*e3),2*(e2*e3-e1*e0);
     -2*(e1*e3-e2*e0),2*(e2*e3+e1*e0),(e3*e3+e0*e0-e2*e2-e1*e1)];

== matlab function qn/11/ODE/A_a ==
  data: u input; V_a output; v input; w input; a output; b output
function [V_a,a,b]= fcn(u,v,w)
V_a=sqrt(u*u+v*v+w*w);
a=atan(w/u);
b=atan(v/V_a);
end

== matlab function qn/11/ODE/F ==
  data: T1 input; F output; T2 input; Tf input; Tp1 input; Tp2 input; Ts1 input; Ts2 input; det1 input; det2 input; det3 input; hg input; lp input; l2 input; l1 input; lt input; ltz input; flag input; F_aav output
function [F,F_aav]  = fcn(T1,T2,Tf,Tp1,Tp2,Ts1,Ts2,det1,det2,det3,hg,lp,l2,l1,lt,ltz,flag)
c=0;
if flag==0
F_uav=[0;
    T1*sin(det1)+ T2*sin(det2);
   -T1*cos(det1)-T2*cos(det2);
   T1*sin(det1)*hg*0.5+ T2*sin(det2)*hg*0.5;
   T1*lp*cos(det1)- T2*lp*cos(det2);
    T1*lp*sin(det1)- T2*lp*sin(det2);];
F_uav_d=[0;0;0;0
    c*(T1*sin(det1)-T2*sin(det2));
    c*(T1*cos(det1)-T2*cos(det2))];
F_aav=[0;0;0;0;0;0];
else if flag==1
F_aav=[Tf*cos(det3);
    Tf*sin(det3);
    -Tp1-Tp2;
    l2*Ts1-l2*Ts2;
    lt*Tp1-lt*Tp2+ltz*Tf*cos(det3);
    l1*Tf*sin(det3)];
F_uav=[0;0;0;0;0;0];
F_uav_d=[0;0;0;0;0;0];
else
    F_aav=flag*[Tf*cos(det3);
    Tf*sin(det3);
    -Tp1-Tp2;
    l2*Ts1-l2*Ts2;
    lt*Tp1-lt*Tp2+ltz*Tf*cos(det3);
    l1*Tf*sin(det3)];
F_uav=(1-flag)*[0;
    T1*sin(det1)+ T2*sin(det2);
   -T1*cos(det1)-T2*cos(det2);
   T1*sin(det1)*hg*0.5+ T2*sin(det2)*hg*0.5;
   T1*lp*cos(det1)- T2*lp*cos(det2);
    T1*lp*sin(det1)- T2*lp*sin(det2);];
F_uav_d=[0;0;0;0;0;0];
end

end
F=F_uav+F_uav_d+F_aav;

== matlab function qn/11/ODE/F1 ==
  data: u input; Fw output; v input; w input; p input; q input; r input; fu input; fv input; fw input; fp input; fq input; fr input; flag input; fu1 input; fv1 input; fw1 input; fp1 input; fq1 input; fr1 input
function Fw  = fcn(u,v,w,p,q,r, fu,fv,fw,fp,fq,fr,flag, fu1,fv1,fw1,fp1,fq1,fr1)
Fw=[-fu*u;
    -fv*v;
    -fw*w;
    -fp*p;
    -fq*q;
    -fr*r];
Fw1=[-fu1*u;
    -fv1*v;
    -fw1*w;
    -fp1*p;
    -fq1*q;
    -fr1*r];
Fw=flag*Fw1+(1-flag)*Fw;

== matlab function qn/11/control/eh uav pd/MATLAB Function9 ==
  data: dx output; ut input; b1 input; x input size=[2 1]; q input; W1 input size=[1 7]; dW1 output; fxp output; w0 input; F1 input
function [dx,dW1,fxp] = fcn(ut,b1,x,q,W1,w0,F1)

%%
h=zeros(1,7);

%%
K1=2*w0;K2=w0*w0;
%  F1=w0^3;
%%
c1=1/3*[-3 -2 -1 0 1 2 3];
c2=2/3*[-3 -2 -1 0 1 2 3];
c=[c1;c2];
b=5;
xp=x';
ye=(q-x(1));
%%
for j=1:1:7
    h(j)=exp(-norm(xp-c(:,j))^2/(2*b^2));
end

k1=0.001;
% k1=0;k2=0;
dW1=F1*h*ye-k1*F1*abs(ye)*W1;

fxp=W1*h';
%%


y=q;
A=[0 1;0 0];
b=[0 1]';
C=[1 0];
K=[K1 K2]';

ye=y-x(1);
D=0;
v=-D*sign(ye);

dx=A*x+b*(fxp+b1*ut-v)+K*(y-C*x);

== matlab function qn/11/ODE/MATLAB Function1 ==
  data: DCM input; F output; g input; h input; flag output
function [F,flag ] = fcn(DCM,g,h)
V0=0.008;
% F=pgV这块是浮力
g=9.8;
a=[0 0.4 0]';
b=[0 -0.4 0]';
y1=DCM*a;
y2=DCM*b;
y1y=[y1(1),y2(1)];
y2y=[y1(2),y2(2)];
xx=[y1(3),y2(3)];
h1=y1(3)+h;
h2=y2(3)+h;
a1=0;
a2=0;
if h1>0 && h2>0
        V=0;
        f=[0 0 0]';
        M=[0 0 0]';
        flag=1;
elseif h1>0 && h2<0
%         a1=interp1(xx,y1y,h,'spline');
%         a2=interp1(xx,y2y,h,'spline');
        V=V0*sqrt((a1-y2(1))^2+(a2-y2(2))^2+(h+y2(3))^2);
        f=[0 0 -1000*g*V]';
        x0=[a1+y2(1) a2+y2(2) h+y2(3)]';
         M= cross(f,x0/2);
         flag=2;

elseif h1<0 && h2>0
%         a1=interp1(xx,y1y,h,'spline');
%         a2=interp1(xx,y2y,h,'spline');
        V=V0*sqrt((a1-y1(1))^2+(a2-y1(2))^2+(h+y1(3))^2);
        f=[0 0 -1000*g*V]';
        x0=[a1+y1(1) a2+y1(2) h+y1(3)]';
         M= cross(f,x0/2);
flag=3;

elseif h1<0 && h2<0
        V=V0*1;
        f=[0 0 -1000*g*V]';
        M=cross(f,y1/2+y2/2);
        flag=4;
else
        V=0;
        f=[0 0 -1000*g*V]';
        M=[0 0 0]';
        flag=5;
end
F=[f;M];

== matlab function qn/11/ODE/Quaternion ==
  data: e0 input size=1; e1 input size=1; new_e0 output; e2 input size=1; e3 input size=1; new_e1 output; new_e2 output; new_e3 output
function [new_e0,new_e1,new_e2,new_e3]= fcn(e0,e1,e2,e3)
e = sqrt(e1*e1+e2*e2+e3*e3+e0*e0);
new_e0=e0/e;
new_e1=e1/e;
new_e2=e2/e;
new_e3=e3/e;

== matlab function qn/11/ODE/Quaternion-Eular ==
  data: e0 input; theta output; e1 input; e2 input; e3 input; pai output; fai output
function [theta,pai,fai]= fcn(e0,e1,e2,e3)
fai=atan2(2*(e0*e1+e2*e3),(e0*e0+e3*e3-e1*e1-e2*e2));%滚转
y=2*(e0*e2-e1*e3);
theta=asin(y);
pai=atan2(2*(e0*e3+e2*e1),(e0*e0+e1*e1-e2*e2-e3*e3));%偏航

== matlab function qn/11/ODE/V_g ==
  data: dx input; X output; dy input; dz input; R output; V_g output; u input
function [X,R,V_g]= fcn(dx,dy,dz,u)
V_g=sqrt(dy*dy+dx*dx);
X=atan2(dy,dx);
R=atan2(dz,sqrt(dx*dx+dy*dy));

== matlab function qn/11/ODE/wind ==
  data: u input; u_r output; v input; w input; u_w input; v_w input; w_w input; v_r output; w_r output
function [u_r,v_r,w_r] = fcn(u,v,w,u_w,v_w,w_w)
u_r=u-u_w;
v_r=v-v_w;
w_r=w-w_w;

== matlab function qn/11/control/MATLAB Function1 ==
  data: uav input; c_uav output; aav input; flag input; c_aav output
function [c_uav,c_aav]= fcn(uav,aav,flag)
if flag==0
c_uav=uav;
c_aav=[0;0;0;0;0;0];
else if flag==1
c_uav=[0;0;0;0];
c_aav=aav;
else
c_aav=aav;
c_uav=uav;
end

end

== matlab function qn/11/control/Subsystem11/MATLAB Function15 ==
  data: flag input; u input; y output
function y = fcn(flag, u)
if flag==1
    y=u* 0;
else
   y= u;
end

== matlab function qn/11/control/Subsystem12/MATLAB Function15 ==
  data: flag input; u input; y output
function y = fcn(flag, u)
if flag==1
    y=u* 0;
else
   y= u;
end

== matlab function qn/11/control/Subsystem13/MATLAB Function17 ==
  data: flag input; u input; y output
function y = fcn(flag, u)
if flag==0
    y= u*0;
else
   y= u;
end
